simulink model "Simulation_testing"  (R2024a)
settings: Solver=VariableStepAuto  StartTime=0.0  StopTime=10.0  RelTol=1e-3
undefined symbols (not defined in the file): R
settings Model: Creator=eduar  LastModifiedBy=eduar

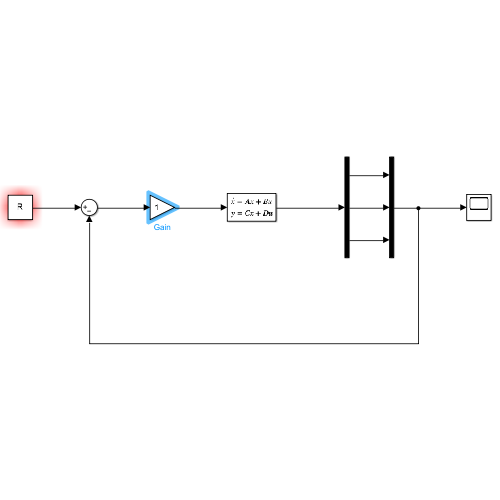
[thumbnail: Simulink's stored preview of the top-level diagram]
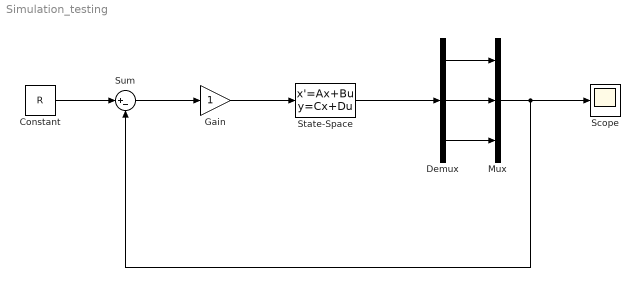
== system Simulation_testing ==
  Constant : Constant  Value=R
  Demux : Demux  Outputs=3
  Gain : Gain
  Mux : Mux  Inputs=3
  Scope : Scope
  State-Space : StateSpace  InitialCondition=0
  Sum : Sum  Inputs=|+-
  wires:
  Constant/1 -> Sum/1
  Sum/1 -> Gain/1
  Gain/1 -> State-Space/1
  State-Space/1 -> Demux/1
  Demux/2 -> Mux/2
  Demux/1 -> Mux/1
  Demux/3 -> Mux/3
  Mux/1 -> Scope/1, Sum/2
